simulink model "BLOM_MPC"  (Simulink 7.4)
settings: Solver=ode1  StartTime=0.0  StopTime=10  FixedStep=dt  MaxStep=1  RelTol=1e-3
values from neighbouring files (symbols this model uses):
  nu = 3    [init_vehicle.m]
  Zcurr = bicycle_fiala_err_discrete(Zcurr,Ufiala,curv,dt,DT_plant,m,mu,Iz,a,b,c,Fz_f,Fz_r,C_f,C_r)    [RunBlomMPC.m]    (also in RunBlomMPC_DT.m)
libraries: BLOM_Lib x10
settings Model: Creator=vichik  LastModifiedBy=Kyle
settings OptimizationCC: InitFltsAndDblsToZero=on
settings DebuggingCC: StrictBusMsg=ErrorLevel1

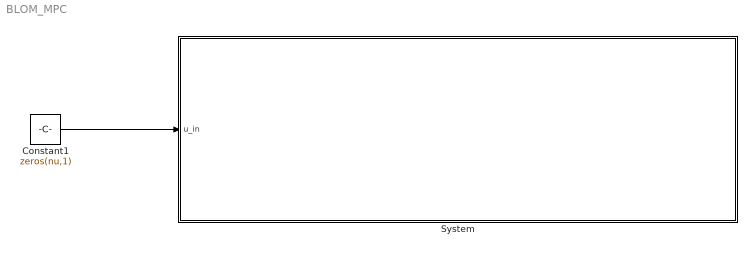
== system BLOM_MPC ==
  Constant1 : Constant  Value=zeros(nu,1)
  System : Subsystem
  wires:
  Constant1/1 -> System/1(u_in)

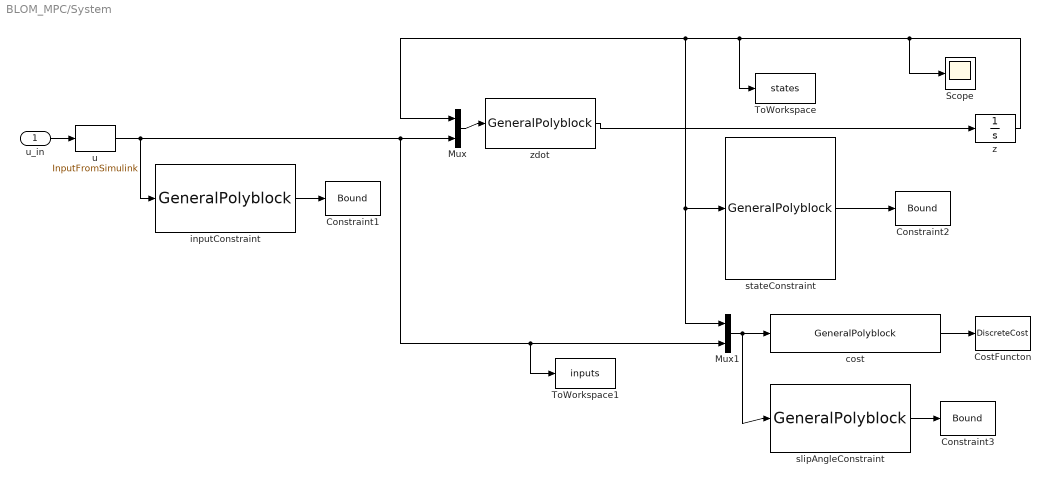
== system BLOM_MPC/System ==
  u_in : Inport
  Constraint1 : BLOM_Lib/Bound  SystemSampleTime=-1  ub=0  lb=-inf  initial_step=on  intermediate_step=on  final_step=on
  Constraint2 : BLOM_Lib/Bound  SystemSampleTime=-1  ub=0  lb=-inf  initial_step=on  intermediate_step=on  final_step=on
  Constraint3 : BLOM_Lib/Bound  SystemSampleTime=-1  ub=0  lb=-inf  initial_step=on  intermediate_step=on  final_step=on
  CostFuncton : BLOM_Lib/DiscreteCost  SystemSampleTime=-1  initial_step=on  intermediate_step=on  final_step=on
  Mux : Mux  Inputs=2
  Mux1 : Mux  Inputs=2
  Scope : Scope
  ToWorkspace : ToWorkspace  VariableName=states  SampleTime=-1  SaveFormat=Structure With Time
  ToWorkspace1 : ToWorkspace  VariableName=inputs  SampleTime=-1  SaveFormat=Structure With Time
  cost : BLOM_Lib/GeneralPolyblock  SystemSampleTime=-1  P_f=cost_f_A  K_f=cost_f_C  P_g=cost_g_A  K_g=cost_g_C  inputs=x_dot, y_dot, psi_dot, e_psi, e_y, s, delta_f, beta_l, beta_r  inputScalar=off  outputScalar=on
  inputConstraint : BLOM_Lib/GeneralPolyblock  SystemSampleTime=-1  P_f=Uconstr_f_A  K_f=Uconstr_f_C  P_g=Uconstr_g_A  K_g=Uconstr_g_C  inputs=delta_f, beta_l, beta_r  inputScalar=off  outputScalar=off
  slipAngleConstraint : BLOM_Lib/GeneralPolyblock  SystemSampleTime=-1  P_f=Sconstr_f_A  K_f=Sconstr_f_C  P_g=Sconstr_g_A  K_g=Sconstr_g_C  inputs=x_dot, y_dot, psi_dot, e_psi, e_y, s, delta_f, beta_l, beta_r  inputScalar=off  outputScalar=off
  stateConstraint : BLOM_Lib/GeneralPolyblock  SystemSampleTime=-1  P_f=Zconstr_f_A  K_f=Zconstr_f_C  P_g=Zconstr_g_A  K_g=Zconstr_g_C  inputs=x_dot, y_dot, psi_dot, e_psi, e_y, s  inputScalar=off  outputScalar=off
  u : BLOM_Lib/InputFromSimulink  SystemSampleTime=-1  interpType=Zero-Order Hold
  z : Integrator  InitialCondition=Zcurr
  zdot : BLOM_Lib/GeneralPolyblock  SystemSampleTime=-1  P_f=zdot_f_A  K_f=zdot_f_C  P_g=zdot_g_A  K_g=zdot_g_C  inputs=x_dot, y_dot, psi_dot, e_psi, e_y, s, delta_f, beta_l, beta_r  inputScalar=off  outputScalar=off
  wires:
  zdot/1 -> z/1
  u/1 -> ToWorkspace1/1, Mux1/2, Mux/2, inputConstraint/1
  stateConstraint/1 -> Constraint2/1
  u_in/1 -> u/1
  inputConstraint/1 -> Constraint1/1
  cost/1 -> CostFuncton/1
  Mux/1 -> zdot/1
  Mux1/1 -> cost/1, slipAngleConstraint/1
  slipAngleConstraint/1 -> Constraint3/1
  z/1 -> Scope/1, ToWorkspace/1, Mux1/1, stateConstraint/1, Mux/1
